simulink model "ChiefMaster_TTC580"  (R2022b)
settings: Solver=FixedStepAuto  StartTime=0.0  StopTime=10  FixedStep=0.01  RelTol=1e-3
values from neighbouring files (symbols this model uses):
  BattBox1_No = single(1)    [Parameters.m]
  BattBox2_No = single(2)    [Parameters.m]
  BattBox3_No = single(3)    [Parameters.m]
  CurrentLB = single(-3)    [Parameters.m]
  CurrentReductionConstant_Lvl0 = single(0.03)    [Parameters.m]
  CurrentReductionConstant_Lvl1 = single(0.05)    [Parameters.m]
  CurrentReductionConstant_Lvl2 = single(0.07)    [Parameters.m]
  CurrentReductionConstant_Lvl3 = single(0.1)    [Parameters.m]
  CurrentUB = single(3)    [Parameters.m]
  DCHV_Minus_In_Delay_ms = single(500)    [Parameters.m]
  FL_sHVC_CellBalanceVoltage_mV = single(3500)    [Parameters.m]
  FL_sInrushCurrent_dividebyzero = single(0.00001)    [Parameters.m]
  FL_u8HMI_BuzzerTimer = uint8(3)    [Parameters.m]
  IP_boActValue = true    [Parameters.m]
  IP_boDeactValue = false    [Parameters.m]
  IP_boInitValue = false    [Parameters.m]
  IP_s_LB = 18000    [Parameters.m]
  IP_s_UB = 22000    [Parameters.m]
  IP_sBatt1_ChargeCurrentMax_Factor = single(0.1)    [Parameters.m]
  IP_sBatt1_ChargeCurrentMax_LB = single(0)    [Parameters.m]
  IP_sBatt1_ChargeCurrentMax_Offset = single(0)    [Parameters.m]
  IP_sBatt1_ChargeCurrentMax_UB = single(6553.5)    [Parameters.m]
  IP_sBatt1_Current_Factor = single(0.1)    [Parameters.m]
  IP_sBatt1_Current_LB = single(-3276.8)    [Parameters.m]
  IP_sBatt1_Current_Offset = single(0)    [Parameters.m]
  IP_sBatt1_Current_UB = single(3276.8)    [Parameters.m]
  IP_sBatt1_DisChargeCurrentMax_Factor = single(0.1)    [Parameters.m]
  IP_sBatt1_DisChargeCurrentMax_LB = single(0)    [Parameters.m]
  IP_sBatt1_DisChargeCurrentMax_Offset = single(0)    [Parameters.m]
  IP_sBatt1_DisChargeCurrentMax_UB = single(6553.5)    [Parameters.m]
  IP_sBatt1_InsulationResistance_Factor = single(5)    [Parameters.m]
  IP_sBatt1_InsulationResistance_LB = single(0)    [Parameters.m]
  IP_sBatt1_InsulationResistance_Offset = single(0)    [Parameters.m]
  IP_sBatt1_InsulationResistance_UB = single(0)    [Parameters.m]
  IP_sBatt1_LiBa_IntResist_mOhm = single(25)    [Parameters.m]
  IP_sBatt1_SOC_Factor = single(1)    [Parameters.m]
  IP_sBatt1_SOC_LB = single(0)    [Parameters.m]
  IP_sBatt1_SOC_Offset = single(0)    [Parameters.m]
  IP_sBatt1_SOC_UB = single(100)    [Parameters.m]
  IP_sBatt1_SOH_Factor = single(1)    [Parameters.m]
  IP_sBatt1_SOH_LB = single(0)    [Parameters.m]
  IP_sBatt1_SOH_Offset = single(0)    [Parameters.m]
  IP_sBatt1_SOH_UB = single(100)    [Parameters.m]
  IP_sBatt1_Ubatt_Factor = single(0.1)    [Parameters.m]
  IP_sBatt1_Ubatt_LB = single(0)    [Parameters.m]
  IP_sBatt1_Ubatt_Offset = single(0)    [Parameters.m]
  IP_sBatt1_Ubatt_UB = single(6553.5)    [Parameters.m]
  IP_sBatt1_UserRi_Factor = single(1)    [Parameters.m]
  IP_sBatt1_UserRi_LB = single(0)    [Parameters.m]
  IP_sBatt1_UserRi_Offset = single(0)    [Parameters.m]
  IP_sBatt1_UserRi_UB = single(255)    [Parameters.m]
  IP_sBatt1_VoltageAtSensor_Factor = single(0.02)    [Parameters.m]
  IP_sBatt1_VoltageAtSensor_LB = single(0)    [Parameters.m]
  IP_sBatt1_VoltageAtSensor_Offset = single(0)    [Parameters.m]
  IP_sBatt1_VoltageAtSensor_UB = single(1310.7)    [Parameters.m]
  IP_sBatt2_LiBa_IntResist_mOhm = single(25)    [Parameters.m]
  IP_sBatt3_LiBa_IntResist_mOhm = single(25)    [Parameters.m]
  IP_sEM_LB = 2000    [Parameters.m]
  IP_sEM_UB = 8000    [Parameters.m]
  IP_sFB_LB = 5000    [Parameters.m]
  IP_sFB_UB = 10000    [Parameters.m]
  IP_sHVIL_LB = 12000    [Parameters.m]
  IP_sHVIL_UB = 15000    [Parameters.m]
  IP_sLoad_Voltage_Factor = single(1)    [Parameters.m]
  IP_sLoad_Voltage_LB = single(0)    [Parameters.m]
  IP_sLoad_Voltage_Offset = single(0)    [Parameters.m]
  IP_sLoad_Voltage_UB = single(65535)    [Parameters.m]
  IP_u8HVIL_Delay_ms = uint8(100)    [Parameters.m]
  IP_u8HW_IN_delay_ms = uint8(100)    [Parameters.m]
  IT_sInsulationSafeValue_kOhm = single(650)    [Parameters.m]
  IT_u8IMD_DelayTime_s = uint8(20)    [Parameters.m]
  MainHV_Minus_In_Delay = single(5)    [Parameters.m]
  MainHV_StatusDelay = single(5)    [Parameters.m]
  NotAvailable_uint16 = single(65535)    [Parameters.m]
  NotAvailable_uint8 = uint8(255)    [Parameters.m]
  OP_boHVIL_Supply = boolean(1)    [Parameters.m]
  SafeCurrentToCloseHV_A = single(5)    [Parameters.m]
  SafeVoltageToCloseHV_V = single(0.5)    [Parameters.m]
  UnexpectedBattChargingFcn_Available = boolean(1)    [Parameters.m]
  Voltage_NA_UB = uint16(65535)    [Parameters.m]
  VoltageSensorAvailableBB1 = boolean(0)    [Parameters.m]
  VoltageSensorAvailableBB2 = boolean(0)    [Parameters.m]
  VoltageSensorAvailableBB3 = boolean(0)    [Parameters.m]
libraries: simulink x184, Library_DataProcessing_v1_1 x167, Library_DataProcessing_v1 x142, libCM x28
(part 16 of 19)

== system ChiefMaster_TTC580/ChiefMaster/Input Processing/LiBa/LiBa_Box1/BMS_CellVoltageNumber/Subsystem2 ==
  byte2 : Inport
  C_LB_CellVoltage02_Timeout : Inport  Port=2
  Bus Creator : BusCreator  Inputs=3
  Constant : Constant  OutDataTypeStr=single
  Constant1 : Constant  Value=0  OutDataTypeStr=single
  Constant2 : Constant  Value=0  OutDataTypeStr=single
  Constant3 : Constant  Value=255  OutDataTypeStr=single
  Constant4 : Constant  Value=0  OutDataTypeStr=single
  Lib_InputProcessing+SafeValueSelector_Data : Library_DataProcessing_v1_1/Lib_InputProcessing+SafeValueSelector_Data  SystemSampleTime=-1  VariantActivationTime=update diagram  Latency=0  AutoFrameSizeCalculation=off
  IP_LB_BMS_ACT_Cel_V_Max_Cel_DataBus : Outport
  wires:
  C_LB_CellVoltage02_Timeout/1 -> Lib_InputProcessing+SafeValueSelector_Data/2
  Bus Creator/1 -> IP_LB_BMS_ACT_Cel_V_Max_Cel_DataBus/1  "IP_LB_BMS_ACT_Cel_V_Max_Cel_DataBus"
  Lib_InputProcessing+SafeValueSelector_Data/1 -> Bus Creator/1
  Constant/1 -> Lib_InputProcessing+SafeValueSelector_Data/3
  Constant4/1 -> Lib_InputProcessing+SafeValueSelector_Data/7, Lib_InputProcessing+SafeValueSelector_Data/8
  Lib_InputProcessing+SafeValueSelector_Data/2 -> Bus Creator/2
  Constant1/1 -> Lib_InputProcessing+SafeValueSelector_Data/4
  byte2/1 -> Lib_InputProcessing+SafeValueSelector_Data/1
  Lib_InputProcessing+SafeValueSelector_Data/3 -> Bus Creator/3
  Constant3/1 -> Lib_InputProcessing+SafeValueSelector_Data/6
  Constant2/1 -> Lib_InputProcessing+SafeValueSelector_Data/5

== system ChiefMaster_TTC580/ChiefMaster/Input Processing/LiBa/LiBa_Box1/BMS_CellVoltageNumber/Subsystem3 ==
  byte3 : Inport
  C_LB_CellVoltage02_Timeout : Inport  Port=2
  Bus Creator : BusCreator  Inputs=3
  Constant : Constant  OutDataTypeStr=single
  Constant1 : Constant  Value=0  OutDataTypeStr=single
  Constant2 : Constant  Value=0  OutDataTypeStr=single
  Constant3 : Constant  Value=255  OutDataTypeStr=single
  Constant4 : Constant  Value=0  OutDataTypeStr=single
  Lib_InputProcessing+SafeValueSelector_Data : Library_DataProcessing_v1_1/Lib_InputProcessing+SafeValueSelector_Data  SystemSampleTime=-1  VariantActivationTime=update diagram  Latency=0  AutoFrameSizeCalculation=off
  IP_LB_BMS_ACT_Cel_V_Max_CMU_DataBus : Outport
  wires:
  Constant2/1 -> Lib_InputProcessing+SafeValueSelector_Data/5
  Constant3/1 -> Lib_InputProcessing+SafeValueSelector_Data/6
  Lib_InputProcessing+SafeValueSelector_Data/3 -> Bus Creator/3
  byte3/1 -> Lib_InputProcessing+SafeValueSelector_Data/1
  Constant1/1 -> Lib_InputProcessing+SafeValueSelector_Data/4
  Lib_InputProcessing+SafeValueSelector_Data/2 -> Bus Creator/2
  Constant4/1 -> Lib_InputProcessing+SafeValueSelector_Data/8, Lib_InputProcessing+SafeValueSelector_Data/7
  Constant/1 -> Lib_InputProcessing+SafeValueSelector_Data/3
  Lib_InputProcessing+SafeValueSelector_Data/1 -> Bus Creator/1
  Bus Creator/1 -> IP_LB_BMS_ACT_Cel_V_Max_CMU_DataBus/1  "IP_LB_BMS_ACT_Cel_V_Max_CMU_DataBus"
  C_LB_CellVoltage02_Timeout/1 -> Lib_InputProcessing+SafeValueSelector_Data/2

== system ChiefMaster_TTC580/ChiefMaster/Input Processing/LiBa/LiBa_Box1/BMS_InsulationMonitor/Subsystem ==
  byte0 : Inport
  byte1 : Inport  Port=2
  C_LB_BMS_InsulationMonitor_Timeout : Inport  Port=3
  Bus Creator : BusCreator  Inputs=3
  Constant : Constant  OutDataTypeStr=single
  Constant1 : Constant  Value=0  OutDataTypeStr=single
  Constant2 : Constant  Value=0  OutDataTypeStr=single
  Constant3 : Constant  Value=65535  OutDataTypeStr=single
  Constant4 : Constant  Value=0  OutDataTypeStr=single
  Lib_2byte_ArthConcat : Library_DataProcessing_v1_1/Lib_2byte_ArthConcat  SystemSampleTime=-1  VariantActivationTime=update diagram  Latency=0  AutoFrameSizeCalculation=off
  Lib_InputProcessing+SafeValueSelector_Data : Library_DataProcessing_v1_1/Lib_InputProcessing+SafeValueSelector_Data  SystemSampleTime=-1  VariantActivationTime=update diagram  Latency=0  AutoFrameSizeCalculation=off
  IP_LB_BMS_Pack_Leak_Pos_Raw_mV_DataBus : Outport
  wires:
  Constant4/1 -> Lib_InputProcessing+SafeValueSelector_Data/7, Lib_InputProcessing+SafeValueSelector_Data/8
  Constant3/1 -> Lib_InputProcessing+SafeValueSelector_Data/6
  Constant2/1 -> Lib_InputProcessing+SafeValueSelector_Data/5
  Constant1/1 -> Lib_InputProcessing+SafeValueSelector_Data/4
  Constant/1 -> Lib_InputProcessing+SafeValueSelector_Data/3
  Bus Creator/1 -> IP_LB_BMS_Pack_Leak_Pos_Raw_mV_DataBus/1  "IP_LB_BMS_Pack_Leak_Pos_Raw_mV_DataBus"
  Lib_InputProcessing+SafeValueSelector_Data/3 -> Bus Creator/3
  Lib_InputProcessing+SafeValueSelector_Data/2 -> Bus Creator/2
  Lib_InputProcessing+SafeValueSelector_Data/1 -> Bus Creator/1
  C_LB_BMS_InsulationMonitor_Timeout/1 -> Lib_InputProcessing+SafeValueSelector_Data/2
  Lib_2byte_ArthConcat/1 -> Lib_InputProcessing+SafeValueSelector_Data/1
  byte1/1 -> Lib_2byte_ArthConcat/2
  byte0/1 -> Lib_2byte_ArthConcat/1

== system ChiefMaster_TTC580/ChiefMaster/Input Processing/LiBa/LiBa_Box1/BMS_InsulationMonitor/Subsystem1 ==
  byte2 : Inport
  byte3 : Inport  Port=2
  C_LB_BMS_InsulationMonitor_Timeout : Inport  Port=3
  Bus Creator : BusCreator  Inputs=3
  Constant : Constant  OutDataTypeStr=single
  Constant1 : Constant  Value=0  OutDataTypeStr=single
  Constant2 : Constant  Value=0  OutDataTypeStr=single
  Constant3 : Constant  Value=65535  OutDataTypeStr=single
  Constant4 : Constant  Value=0  OutDataTypeStr=single
  Lib_2byte_ArthConcat : Library_DataProcessing_v1_1/Lib_2byte_ArthConcat  SystemSampleTime=-1  VariantActivationTime=update diagram  Latency=0  AutoFrameSizeCalculation=off
  Lib_InputProcessing+SafeValueSelector_Data : Library_DataProcessing_v1_1/Lib_InputProcessing+SafeValueSelector_Data  SystemSampleTime=-1  VariantActivationTime=update diagram  Latency=0  AutoFrameSizeCalculation=off
  IP_LB_BMS_Pack_Leak_Neg_Raw_mV_DataBus : Outport
  wires:
  Bus Creator/1 -> IP_LB_BMS_Pack_Leak_Neg_Raw_mV_DataBus/1  "IP_LB_BMS_Pack_Leak_Neg_Raw_mV_DataBus"
  C_LB_BMS_InsulationMonitor_Timeout/1 -> Lib_InputProcessing+SafeValueSelector_Data/2
  byte3/1 -> Lib_2byte_ArthConcat/2
  byte2/1 -> Lib_2byte_ArthConcat/1
  Constant3/1 -> Lib_InputProcessing+SafeValueSelector_Data/6
  Constant2/1 -> Lib_InputProcessing+SafeValueSelector_Data/5
  Lib_InputProcessing+SafeValueSelector_Data/3 -> Bus Creator/3
  Lib_InputProcessing+SafeValueSelector_Data/2 -> Bus Creator/2
  Constant/1 -> Lib_InputProcessing+SafeValueSelector_Data/3
  Lib_InputProcessing+SafeValueSelector_Data/1 -> Bus Creator/1
  Constant1/1 -> Lib_InputProcessing+SafeValueSelector_Data/4
  Lib_2byte_ArthConcat/1 -> Lib_InputProcessing+SafeValueSelector_Data/1
  Constant4/1 -> Lib_InputProcessing+SafeValueSelector_Data/7, Lib_InputProcessing+SafeValueSelector_Data/8

== system ChiefMaster_TTC580/ChiefMaster/Input Processing/LiBa/LiBa_Box1/BMS_InsulationMonitor/Subsystem2 ==
  byte4 : Inport
  byte5 : Inport  Port=2
  C_LB_BMS_InsulationMonitor_Timeout : Inport  Port=3
  Bus Creator : BusCreator  Inputs=3
  Constant : Constant  OutDataTypeStr=single
  Constant1 : Constant  Value=0  OutDataTypeStr=single
  Constant2 : Constant  Value=0  OutDataTypeStr=single
  Constant3 : Constant  Value=65535  OutDataTypeStr=single
  Constant4 : Constant  Value=0  OutDataTypeStr=single
  Lib_2byte_ArthConcat : Library_DataProcessing_v1_1/Lib_2byte_ArthConcat  SystemSampleTime=-1  VariantActivationTime=update diagram  Latency=0  AutoFrameSizeCalculation=off
  Lib_InputProcessing+SafeValueSelector_Data : Library_DataProcessing_v1_1/Lib_InputProcessing+SafeValueSelector_Data  SystemSampleTime=-1  VariantActivationTime=update diagram  Latency=0  AutoFrameSizeCalculation=off
  IP_LB_BMS_Pack_Leak_Mid_Raw_mV_DataBus : Outport
  wires:
  byte5/1 -> Lib_2byte_ArthConcat/2
  byte4/1 -> Lib_2byte_ArthConcat/1
  C_LB_BMS_InsulationMonitor_Timeout/1 -> Lib_InputProcessing+SafeValueSelector_Data/2
  Bus Creator/1 -> IP_LB_BMS_Pack_Leak_Mid_Raw_mV_DataBus/1  "IP_LB_BMS_Pack_Leak_Mid_Raw_mV_DataBus"
  Lib_InputProcessing+SafeValueSelector_Data/1 -> Bus Creator/1
  Constant/1 -> Lib_InputProcessing+SafeValueSelector_Data/3
  Constant4/1 -> Lib_InputProcessing+SafeValueSelector_Data/7, Lib_InputProcessing+SafeValueSelector_Data/8
  Lib_InputProcessing+SafeValueSelector_Data/2 -> Bus Creator/2
  Constant1/1 -> Lib_InputProcessing+SafeValueSelector_Data/4
  Lib_2byte_ArthConcat/1 -> Lib_InputProcessing+SafeValueSelector_Data/1
  Lib_InputProcessing+SafeValueSelector_Data/3 -> Bus Creator/3
  Constant3/1 -> Lib_InputProcessing+SafeValueSelector_Data/6
  Constant2/1 -> Lib_InputProcessing+SafeValueSelector_Data/5

== system ChiefMaster_TTC580/ChiefMaster/Input Processing/LiBa/LiBa_Box1/BMS_Status01/Subsystem1 ==
  byte1 : Inport
  C_LB_BMS_Status01_Timeout : Inport  Port=2
  Bus Creator : BusCreator  Inputs=3
  Constant : Constant  OutDataTypeStr=single
  Constant1 : Constant  Value=0  OutDataTypeStr=single
  Constant2 : Constant  Value=0  OutDataTypeStr=single
  Constant3 : Constant  Value=255  OutDataTypeStr=single
  Constant4 : Constant  Value=0  OutDataTypeStr=single
  Lib_InputProcessing+SafeValueSelector_Data : Library_DataProcessing_v1_1/Lib_InputProcessing+SafeValueSelector_Data  SystemSampleTime=-1  VariantActivationTime=update diagram  Latency=0  AutoFrameSizeCalculation=off
  IP_LB_BMS_IO_state_Input_DataBus : Outport
  wires:
  byte1/1 -> Lib_InputProcessing+SafeValueSelector_Data/1
  Bus Creator/1 -> IP_LB_BMS_IO_state_Input_DataBus/1  "IP_LB_BMS_IO_state_Input_DataBus"
  C_LB_BMS_Status01_Timeout/1 -> Lib_InputProcessing+SafeValueSelector_Data/2
  Constant3/1 -> Lib_InputProcessing+SafeValueSelector_Data/6
  Constant2/1 -> Lib_InputProcessing+SafeValueSelector_Data/5
  Lib_InputProcessing+SafeValueSelector_Data/3 -> Bus Creator/3
  Lib_InputProcessing+SafeValueSelector_Data/2 -> Bus Creator/2
  Constant/1 -> Lib_InputProcessing+SafeValueSelector_Data/3
  Lib_InputProcessing+SafeValueSelector_Data/1 -> Bus Creator/1
  Constant1/1 -> Lib_InputProcessing+SafeValueSelector_Data/4
  Constant4/1 -> Lib_InputProcessing+SafeValueSelector_Data/7, Lib_InputProcessing+SafeValueSelector_Data/8

== system ChiefMaster_TTC580/ChiefMaster/Input Processing/LiBa/LiBa_Box1/BMS_Status01/Subsystem2 ==
  byte2 : Inport
  C_LB_BMS_Status01_Timeout : Inport  Port=2
  Bus Creator : BusCreator  Inputs=3
  Constant : Constant  OutDataTypeStr=single
  Constant1 : Constant  Value=0  OutDataTypeStr=single
  Constant2 : Constant  Value=0  OutDataTypeStr=single
  Constant3 : Constant  Value=255  OutDataTypeStr=single
  Constant4 : Constant  Value=0  OutDataTypeStr=single
  Lib_InputProcessing+SafeValueSelector_Data : Library_DataProcessing_v1_1/Lib_InputProcessing+SafeValueSelector_Data  SystemSampleTime=-1  VariantActivationTime=update diagram  Latency=0  AutoFrameSizeCalculation=off
  IP_LB_BMS_IO_State_Output_DataBus : Outport
  wires:
  byte2/1 -> Lib_InputProcessing+SafeValueSelector_Data/1
  C_LB_BMS_Status01_Timeout/1 -> Lib_InputProcessing+SafeValueSelector_Data/2
  Bus Creator/1 -> IP_LB_BMS_IO_State_Output_DataBus/1  "IP_LB_BMS_IO_State_Output_DataBus"
  Lib_InputProcessing+SafeValueSelector_Data/1 -> Bus Creator/1
  Constant/1 -> Lib_InputProcessing+SafeValueSelector_Data/3
  Constant4/1 -> Lib_InputProcessing+SafeValueSelector_Data/7, Lib_InputProcessing+SafeValueSelector_Data/8
  Lib_InputProcessing+SafeValueSelector_Data/2 -> Bus Creator/2
  Constant1/1 -> Lib_InputProcessing+SafeValueSelector_Data/4
  Lib_InputProcessing+SafeValueSelector_Data/3 -> Bus Creator/3
  Constant3/1 -> Lib_InputProcessing+SafeValueSelector_Data/6
  Constant2/1 -> Lib_InputProcessing+SafeValueSelector_Data/5

== system ChiefMaster_TTC580/ChiefMaster/Input Processing/LiBa/LiBa_Box1/BMS_Status01/Subsystem3 ==
  byte4 : Inport
  byte5 : Inport  Port=2
  C_LB_BMS_Status01_Timeout : Inport  Port=3
  Bus Creator : BusCreator  Inputs=3
  Constant : Constant  Value=0.1  OutDataTypeStr=single
  Constant1 : Constant  Value=0  OutDataTypeStr=single
  Constant2 : Constant  Value=0  OutDataTypeStr=single
  Constant3 : Constant  Value=6553.5  OutDataTypeStr=single
  Constant4 : Constant  Value=0  OutDataTypeStr=single
  Lib_2byte_ArthConcat : Library_DataProcessing_v1_1/Lib_2byte_ArthConcat  SystemSampleTime=-1  VariantActivationTime=update diagram  Latency=0  AutoFrameSizeCalculation=off
  Lib_InputProcessing+SafeValueSelector_Data : Library_DataProcessing_v1_1/Lib_InputProcessing+SafeValueSelector_Data  SystemSampleTime=-1  VariantActivationTime=update diagram  Latency=0  AutoFrameSizeCalculation=off
  IP_LB_BMS_DYN_Lim_Current_IN_A_DataBus : Outport
  wires:
  Bus Creator/1 -> IP_LB_BMS_DYN_Lim_Current_IN_A_DataBus/1  "IP_LB_BMS_DYN_Lim_Current_IN_A_DataBus"
  Constant3/1 -> Lib_InputProcessing+SafeValueSelector_Data/6
  Lib_2byte_ArthConcat/1 -> Lib_InputProcessing+SafeValueSelector_Data/1
  Constant1/1 -> Lib_InputProcessing+SafeValueSelector_Data/4
  Constant4/1 -> Lib_InputProcessing+SafeValueSelector_Data/8, Lib_InputProcessing+SafeValueSelector_Data/7
  Constant/1 -> Lib_InputProcessing+SafeValueSelector_Data/3
  Constant2/1 -> Lib_InputProcessing+SafeValueSelector_Data/5
  Lib_InputProcessing+SafeValueSelector_Data/1 -> Bus Creator/1
  Lib_InputProcessing+SafeValueSelector_Data/3 -> Bus Creator/3
  Lib_InputProcessing+SafeValueSelector_Data/2 -> Bus Creator/2
  byte4/1 -> Lib_2byte_ArthConcat/1
  byte5/1 -> Lib_2byte_ArthConcat/2
  C_LB_BMS_Status01_Timeout/1 -> Lib_InputProcessing+SafeValueSelector_Data/2

== system ChiefMaster_TTC580/ChiefMaster/Input Processing/LiBa/LiBa_Box1/BMS_Status01/Subsystem4 ==
  byte6 : Inport
  byte7 : Inport  Port=2
  C_LB_BMS_Status01_Timeout : Inport  Port=3
  Bus Creator : BusCreator  Inputs=3
  Constant : Constant  Value=0.1  OutDataTypeStr=single
  Constant1 : Constant  Value=0  OutDataTypeStr=single
  Constant2 : Constant  Value=0  OutDataTypeStr=single
  Constant3 : Constant  Value=6553.5  OutDataTypeStr=single
  Constant4 : Constant  Value=0  OutDataTypeStr=single
  Lib_2byte_ArthConcat : Library_DataProcessing_v1_1/Lib_2byte_ArthConcat  SystemSampleTime=-1  VariantActivationTime=update diagram  Latency=0  AutoFrameSizeCalculation=off
  Lib_InputProcessing+SafeValueSelector_Data : Library_DataProcessing_v1_1/Lib_InputProcessing+SafeValueSelector_Data  SystemSampleTime=-1  VariantActivationTime=update diagram  Latency=0  AutoFrameSizeCalculation=off
  IP_LB_BMS_DYN_Lim_Current_OUT_A_DataBus : Outport
  wires:
  C_LB_BMS_Status01_Timeout/1 -> Lib_InputProcessing+SafeValueSelector_Data/2
  byte7/1 -> Lib_2byte_ArthConcat/2
  byte6/1 -> Lib_2byte_ArthConcat/1
  Lib_InputProcessing+SafeValueSelector_Data/2 -> Bus Creator/2
  Lib_InputProcessing+SafeValueSelector_Data/3 -> Bus Creator/3
  Lib_InputProcessing+SafeValueSelector_Data/1 -> Bus Creator/1
  Constant2/1 -> Lib_InputProcessing+SafeValueSelector_Data/5
  Constant/1 -> Lib_InputProcessing+SafeValueSelector_Data/3
  Constant4/1 -> Lib_InputProcessing+SafeValueSelector_Data/7, Lib_InputProcessing+SafeValueSelector_Data/8
  Constant1/1 -> Lib_InputProcessing+SafeValueSelector_Data/4
  Lib_2byte_ArthConcat/1 -> Lib_InputProcessing+SafeValueSelector_Data/1
  Constant3/1 -> Lib_InputProcessing+SafeValueSelector_Data/6
  Bus Creator/1 -> IP_LB_BMS_DYN_Lim_Current_OUT_A_DataBus/1  "IP_LB_BMS_DYN_Lim_Current_OUT_A_DataBus"

== system ChiefMaster_TTC580/ChiefMaster/Input Processing/LiBa/LiBa_Box1/BMS_Status02/Subsystem1 ==
  byte2 : Inport
  byte3 : Inport  Port=2
  byte4 : Inport  Port=3
  byte5 : Inport  Port=4
  C_LB_BMS_Status02_Timeout : Inport  Port=5
  Bus Creator : BusCreator  Inputs=3
  Constant : Constant  Value=0.01  OutDataTypeStr=single
  Constant1 : Constant  Value=0  OutDataTypeStr=single
  Constant2 : Constant  Value=-21474836.48  OutDataTypeStr=single
  Constant3 : Constant  Value=21474836.47  OutDataTypeStr=single
  Constant4 : Constant  Value=0  OutDataTypeStr=single
  Data Type Conversion : DataTypeConversion  OutDataTypeStr=int32  SaturateOnIntegerOverflow=off  RndMeth=Floor
  Lib_4byte_ArthConcat : Library_DataProcessing_v1_1/Lib_4byte_ArthConcat  SystemSampleTime=-1  VariantActivationTime=update diagram  Latency=0  AutoFrameSizeCalculation=off
  Lib_InputProcessing+SafeValueSelector_Data : Library_DataProcessing_v1_1/Lib_InputProcessing+SafeValueSelector_Data  SystemSampleTime=-1  VariantActivationTime=update diagram  Latency=0  AutoFrameSizeCalculation=off
  IP_LB_BMS_Pack_Current_Master_mA_DataBus : Outport
  wires:
  Data Type Conversion/1 -> Lib_InputProcessing+SafeValueSelector_Data/1
  Bus Creator/1 -> IP_LB_BMS_Pack_Current_Master_mA_DataBus/1  "IP_LB_BMS_Pack_Current_Master_mA_DataBus"
  Constant3/1 -> Lib_InputProcessing+SafeValueSelector_Data/6
  Lib_4byte_ArthConcat/1 -> Data Type Conversion/1
  Constant1/1 -> Lib_InputProcessing+SafeValueSelector_Data/4
  Constant4/1 -> Lib_InputProcessing+SafeValueSelector_Data/8, Lib_InputProcessing+SafeValueSelector_Data/7
  Constant/1 -> Lib_InputProcessing+SafeValueSelector_Data/3
  Constant2/1 -> Lib_InputProcessing+SafeValueSelector_Data/5
  Lib_InputProcessing+SafeValueSelector_Data/1 -> Bus Creator/1
  Lib_InputProcessing+SafeValueSelector_Data/3 -> Bus Creator/3
  Lib_InputProcessing+SafeValueSelector_Data/2 -> Bus Creator/2
  byte2/1 -> Lib_4byte_ArthConcat/1
  byte3/1 -> Lib_4byte_ArthConcat/2
  C_LB_BMS_Status02_Timeout/1 -> Lib_InputProcessing+SafeValueSelector_Data/2
  byte4/1 -> Lib_4byte_ArthConcat/3
  byte5/1 -> Lib_4byte_ArthConcat/4

== system ChiefMaster_TTC580/ChiefMaster/Input Processing/LiBa/LiBa_Box1/BMS_Status02/Subsystem2 ==
  byte6 : Inport
  byte7 : Inport  Port=2
  C_LB_BMS_Status02_Timeout : Inport  Port=3
  Bus Creator : BusCreator  Inputs=3
  Constant : Constant  Value=0.1  OutDataTypeStr=single
  Constant1 : Constant  Value=0  OutDataTypeStr=single
  Constant2 : Constant  Value=0  OutDataTypeStr=single
  Constant3 : Constant  Value=6553.5  OutDataTypeStr=single
  Constant4 : Constant  Value=0  OutDataTypeStr=single
  Lib_2byte_ArthConcat : Library_DataProcessing_v1_1/Lib_2byte_ArthConcat  SystemSampleTime=-1  VariantActivationTime=update diagram  Latency=0  AutoFrameSizeCalculation=off
  Lib_InputProcessing+SafeValueSelector_Data : Library_DataProcessing_v1_1/Lib_InputProcessing+SafeValueSelector_Data  SystemSampleTime=-1  VariantActivationTime=update diagram  Latency=0  AutoFrameSizeCalculation=off
  IP_LB_BMS_Pack_V_Cells_DataBus : Outport
  wires:
  Lib_2byte_ArthConcat/1 -> Lib_InputProcessing+SafeValueSelector_Data/1
  Bus Creator/1 -> IP_LB_BMS_Pack_V_Cells_DataBus/1  "IP_LB_BMS_Pack_V_Cells_DataBus"
  Constant3/1 -> Lib_InputProcessing+SafeValueSelector_Data/6
  Constant1/1 -> Lib_InputProcessing+SafeValueSelector_Data/4
  Constant4/1 -> Lib_InputProcessing+SafeValueSelector_Data/8, Lib_InputProcessing+SafeValueSelector_Data/7
  Constant/1 -> Lib_InputProcessing+SafeValueSelector_Data/3
  Constant2/1 -> Lib_InputProcessing+SafeValueSelector_Data/5
  Lib_InputProcessing+SafeValueSelector_Data/1 -> Bus Creator/1
  Lib_InputProcessing+SafeValueSelector_Data/3 -> Bus Creator/3
  Lib_InputProcessing+SafeValueSelector_Data/2 -> Bus Creator/2
  byte6/1 -> Lib_2byte_ArthConcat/1
  byte7/1 -> Lib_2byte_ArthConcat/2
  C_LB_BMS_Status02_Timeout/1 -> Lib_InputProcessing+SafeValueSelector_Data/2

== system ChiefMaster_TTC580/ChiefMaster/Input Processing/LiBa/LiBa_Box1/BMS_Status02/Subsystem3 ==
  byte0 : Inport
  byte1 : Inport  Port=2
  C_LB_BMS_Status02_Timeout : Inport  Port=3
  Bus Creator : BusCreator  Inputs=3
  Constant : Constant  Value=0.01  OutDataTypeStr=single
  Constant1 : Constant  Value=0  OutDataTypeStr=single
  Constant2 : Constant  Value=-327.68  OutDataTypeStr=single
  Constant3 : Constant  Value=327.67  OutDataTypeStr=single
  Constant4 : Constant  Value=0  OutDataTypeStr=single
  Data Type Conversion : DataTypeConversion  OutDataTypeStr=int16  SaturateOnIntegerOverflow=off  RndMeth=Floor
  Lib_2byte_ArthConcat : Library_DataProcessing_v1_1/Lib_2byte_ArthConcat  SystemSampleTime=-1  VariantActivationTime=update diagram  Latency=0  AutoFrameSizeCalculation=off
  Lib_InputProcessing+SafeValueSelector_Data : Library_DataProcessing_v1_1/Lib_InputProcessing+SafeValueSelector_Data  SystemSampleTime=-1  VariantActivationTime=update diagram  Latency=0  AutoFrameSizeCalculation=off
  IP_LB_BMS_Pack_Q_SOC_Internal_DataBus : Outport
  wires:
  C_LB_BMS_Status02_Timeout/1 -> Lib_InputProcessing+SafeValueSelector_Data/2
  byte1/1 -> Lib_2byte_ArthConcat/2
  byte0/1 -> Lib_2byte_ArthConcat/1
  Lib_InputProcessing+SafeValueSelector_Data/2 -> Bus Creator/2
  Lib_InputProcessing+SafeValueSelector_Data/3 -> Bus Creator/3
  Lib_InputProcessing+SafeValueSelector_Data/1 -> Bus Creator/1
  Constant2/1 -> Lib_InputProcessing+SafeValueSelector_Data/5
  Constant/1 -> Lib_InputProcessing+SafeValueSelector_Data/3
  Constant4/1 -> Lib_InputProcessing+SafeValueSelector_Data/7, Lib_InputProcessing+SafeValueSelector_Data/8
  Constant1/1 -> Lib_InputProcessing+SafeValueSelector_Data/4
  Lib_2byte_ArthConcat/1 -> Data Type Conversion/1
  Constant3/1 -> Lib_InputProcessing+SafeValueSelector_Data/6
  Bus Creator/1 -> IP_LB_BMS_Pack_Q_SOC_Internal_DataBus/1  "IP_LB_BMS_Pack_Q_SOC_Internal_DataBus"
  Data Type Conversion/1 -> Lib_InputProcessing+SafeValueSelector_Data/1

== system ChiefMaster_TTC580/ChiefMaster/Input Processing/LiBa/LiBa_Box1/BMS_Status03/Subsystem3 ==
  byte0 : Inport
  byte1 : Inport  Port=2
  C_LB_BMS_Status03_Timeout : Inport  Port=3
  Bus Creator : BusCreator  Inputs=3
  Constant : Constant  Value=0.1  OutDataTypeStr=single
  Constant1 : Constant  Value=0  OutDataTypeStr=single
  Constant2 : Constant  Value=0  OutDataTypeStr=single
  Constant3 : Constant  Value=6553.5  OutDataTypeStr=single
  Constant4 : Constant  Value=0  OutDataTypeStr=single
  Lib_2byte_ArthConcat : Library_DataProcessing_v1_1/Lib_2byte_ArthConcat  SystemSampleTime=-1  VariantActivationTime=update diagram  Latency=0  AutoFrameSizeCalculation=off
  Lib_InputProcessing+SafeValueSelector_Data : Library_DataProcessing_v1_1/Lib_InputProcessing+SafeValueSelector_Data  SystemSampleTime=-1  VariantActivationTime=update diagram  Latency=0  AutoFrameSizeCalculation=off
  IP_LB_BMS_REQ_Charger_Current_A_DataBus : Outport
  wires:
  Lib_2byte_ArthConcat/1 -> Lib_InputProcessing+SafeValueSelector_Data/1
  Bus Creator/1 -> IP_LB_BMS_REQ_Charger_Current_A_DataBus/1  "IP_LB_BMS_REQ_Charger_Current_A_DataBus"
  Constant3/1 -> Lib_InputProcessing+SafeValueSelector_Data/6
  Constant1/1 -> Lib_InputProcessing+SafeValueSelector_Data/4
  Constant4/1 -> Lib_InputProcessing+SafeValueSelector_Data/8, Lib_InputProcessing+SafeValueSelector_Data/7
  Constant/1 -> Lib_InputProcessing+SafeValueSelector_Data/3
  Constant2/1 -> Lib_InputProcessing+SafeValueSelector_Data/5
  Lib_InputProcessing+SafeValueSelector_Data/1 -> Bus Creator/1
  Lib_InputProcessing+SafeValueSelector_Data/3 -> Bus Creator/3
  Lib_InputProcessing+SafeValueSelector_Data/2 -> Bus Creator/2
  byte0/1 -> Lib_2byte_ArthConcat/1
  byte1/1 -> Lib_2byte_ArthConcat/2
  C_LB_BMS_Status03_Timeout/1 -> Lib_InputProcessing+SafeValueSelector_Data/2

== system ChiefMaster_TTC580/ChiefMaster/Input Processing/LiBa/LiBa_Box2/BMS_CellTemperature/Subsystem ==
  byte0 : Inport
  C_LB_BMS_CellTemperature_Timeout : Inport  Port=2
  Bus Creator : BusCreator  Inputs=3
  Constant : Constant  OutDataTypeStr=single
  Constant1 : Constant  Value=0  OutDataTypeStr=single
  Constant2 : Constant  Value=-128  OutDataTypeStr=single
  Constant3 : Constant  Value=127  OutDataTypeStr=single
  Constant4 : Constant  Value=0  OutDataTypeStr=single
  Data Type Conversion : DataTypeConversion  OutDataTypeStr=int8  SaturateOnIntegerOverflow=off  RndMeth=Floor
  Lib_InputProcessing+SafeValueSelector_Data : Library_DataProcessing_v1_1/Lib_InputProcessing+SafeValueSelector_Data  SystemSampleTime=-1  VariantActivationTime=update diagram  Latency=0  AutoFrameSizeCalculation=off
  IP_LB_BMS_ACT_Cel_T_Avg_DataBus : Outport
  wires:
  byte0/1 -> Data Type Conversion/1
  C_LB_BMS_CellTemperature_Timeout/1 -> Lib_InputProcessing+SafeValueSelector_Data/2
  Lib_InputProcessing+SafeValueSelector_Data/1 -> Bus Creator/1
  Lib_InputProcessing+SafeValueSelector_Data/2 -> Bus Creator/2
  Lib_InputProcessing+SafeValueSelector_Data/3 -> Bus Creator/3
  Bus Creator/1 -> IP_LB_BMS_ACT_Cel_T_Avg_DataBus/1  "IP_LB_BMS_ACT_Cel_T_Avg_DataBus"
  Constant/1 -> Lib_InputProcessing+SafeValueSelector_Data/3
  Constant1/1 -> Lib_InputProcessing+SafeValueSelector_Data/4
  Constant2/1 -> Lib_InputProcessing+SafeValueSelector_Data/5
  Constant3/1 -> Lib_InputProcessing+SafeValueSelector_Data/6
  Constant4/1 -> Lib_InputProcessing+SafeValueSelector_Data/8, Lib_InputProcessing+SafeValueSelector_Data/7
  Data Type Conversion/1 -> Lib_InputProcessing+SafeValueSelector_Data/1

== system ChiefMaster_TTC580/ChiefMaster/Input Processing/LiBa/LiBa_Box2/BMS_CellTemperature/Subsystem1 ==
  byte1 : Inport
  C_LB_BMS_CellTemperature_Timeout : Inport  Port=2
  Bus Creator : BusCreator  Inputs=3
  Constant : Constant  OutDataTypeStr=single
  Constant1 : Constant  Value=0  OutDataTypeStr=single
  Constant2 : Constant  Value=-128  OutDataTypeStr=single
  Constant3 : Constant  Value=127  OutDataTypeStr=single
  Constant4 : Constant  Value=0  OutDataTypeStr=single
  Data Type Conversion : DataTypeConversion  OutDataTypeStr=int8  SaturateOnIntegerOverflow=off  RndMeth=Floor
  Lib_InputProcessing+SafeValueSelector_Data : Library_DataProcessing_v1_1/Lib_InputProcessing+SafeValueSelector_Data  SystemSampleTime=-1  VariantActivationTime=update diagram  Latency=0  AutoFrameSizeCalculation=off
  IP_LB_BMS_ACT_Cel_T_Min_Value_DataBus : Outport
  wires:
  Constant4/1 -> Lib_InputProcessing+SafeValueSelector_Data/8, Lib_InputProcessing+SafeValueSelector_Data/7
  byte1/1 -> Data Type Conversion/1
  Constant1/1 -> Lib_InputProcessing+SafeValueSelector_Data/4
  Lib_InputProcessing+SafeValueSelector_Data/1 -> Bus Creator/1
  Constant/1 -> Lib_InputProcessing+SafeValueSelector_Data/3
  Lib_InputProcessing+SafeValueSelector_Data/2 -> Bus Creator/2
  Lib_InputProcessing+SafeValueSelector_Data/3 -> Bus Creator/3
  Constant2/1 -> Lib_InputProcessing+SafeValueSelector_Data/5
  Constant3/1 -> Lib_InputProcessing+SafeValueSelector_Data/6
  C_LB_BMS_CellTemperature_Timeout/1 -> Lib_InputProcessing+SafeValueSelector_Data/2
  Bus Creator/1 -> IP_LB_BMS_ACT_Cel_T_Min_Value_DataBus/1  "IP_LB_BMS_ACT_Cel_T_Min_Value_DataBus"
  Data Type Conversion/1 -> Lib_InputProcessing+SafeValueSelector_Data/1

== system ChiefMaster_TTC580/ChiefMaster/Input Processing/LiBa/LiBa_Box2/BMS_CellTemperature/Subsystem2 ==
  byte2 : Inport
  C_LB_BMS_CellTemperature_Timeout : Inport  Port=2
  Bus Creator : BusCreator  Inputs=3
  Constant : Constant  OutDataTypeStr=single
  Constant1 : Constant  Value=0  OutDataTypeStr=single
  Constant2 : Constant  Value=-128  OutDataTypeStr=single
  Constant3 : Constant  Value=127  OutDataTypeStr=single
  Constant4 : Constant  Value=0  OutDataTypeStr=single
  Data Type Conversion : DataTypeConversion  OutDataTypeStr=int8  SaturateOnIntegerOverflow=off  RndMeth=Floor
  Lib_InputProcessing+SafeValueSelector_Data : Library_DataProcessing_v1_1/Lib_InputProcessing+SafeValueSelector_Data  SystemSampleTime=-1  VariantActivationTime=update diagram  Latency=0  AutoFrameSizeCalculation=off
  IP_LB_BMS_ACT_Cel_T_Max_Value_DataBus : Outport
  wires:
  Constant2/1 -> Lib_InputProcessing+SafeValueSelector_Data/5
  Constant3/1 -> Lib_InputProcessing+SafeValueSelector_Data/6
  Lib_InputProcessing+SafeValueSelector_Data/3 -> Bus Creator/3
  byte2/1 -> Data Type Conversion/1
  Constant1/1 -> Lib_InputProcessing+SafeValueSelector_Data/4
  Lib_InputProcessing+SafeValueSelector_Data/2 -> Bus Creator/2
  Constant4/1 -> Lib_InputProcessing+SafeValueSelector_Data/8, Lib_InputProcessing+SafeValueSelector_Data/7
  Constant/1 -> Lib_InputProcessing+SafeValueSelector_Data/3
  Lib_InputProcessing+SafeValueSelector_Data/1 -> Bus Creator/1
  Bus Creator/1 -> IP_LB_BMS_ACT_Cel_T_Max_Value_DataBus/1  "IP_LB_BMS_ACT_Cel_T_Max_Value_DataBus"
  C_LB_BMS_CellTemperature_Timeout/1 -> Lib_InputProcessing+SafeValueSelector_Data/2
  Data Type Conversion/1 -> Lib_InputProcessing+SafeValueSelector_Data/1

== system ChiefMaster_TTC580/ChiefMaster/Input Processing/LiBa/LiBa_Box2/BMS_CellTemperature/Subsystem3 ==
  byte3 : Inport
  C_LB_BMS_CellTemperature_Timeout : Inport  Port=2
  Bus Creator : BusCreator  Inputs=3
  Constant : Constant  OutDataTypeStr=single
  Constant1 : Constant  Value=0  OutDataTypeStr=single
  Constant2 : Constant  Value=0  OutDataTypeStr=single
  Constant3 : Constant  Value=255  OutDataTypeStr=single
  Constant4 : Constant  Value=0  OutDataTypeStr=single
  Lib_InputProcessing+SafeValueSelector_Data : Library_DataProcessing_v1_1/Lib_InputProcessing+SafeValueSelector_Data  SystemSampleTime=-1  VariantActivationTime=update diagram  Latency=0  AutoFrameSizeCalculation=off
  IP_LB_BMS_ACT_Cel_T_Min_Cel_DataBus : Outport
  wires:
  C_LB_BMS_CellTemperature_Timeout/1 -> Lib_InputProcessing+SafeValueSelector_Data/2
  Bus Creator/1 -> IP_LB_BMS_ACT_Cel_T_Min_Cel_DataBus/1  "IP_LB_BMS_ACT_Cel_T_Min_Cel_DataBus"
  Lib_InputProcessing+SafeValueSelector_Data/1 -> Bus Creator/1
  Constant/1 -> Lib_InputProcessing+SafeValueSelector_Data/3
  Constant4/1 -> Lib_InputProcessing+SafeValueSelector_Data/7, Lib_InputProcessing+SafeValueSelector_Data/8
  Lib_InputProcessing+SafeValueSelector_Data/2 -> Bus Creator/2
  Constant1/1 -> Lib_InputProcessing+SafeValueSelector_Data/4
  byte3/1 -> Lib_InputProcessing+SafeValueSelector_Data/1
  Lib_InputProcessing+SafeValueSelector_Data/3 -> Bus Creator/3
  Constant3/1 -> Lib_InputProcessing+SafeValueSelector_Data/6
  Constant2/1 -> Lib_InputProcessing+SafeValueSelector_Data/5

== system ChiefMaster_TTC580/ChiefMaster/Input Processing/LiBa/LiBa_Box2/BMS_CellTemperature/Subsystem4 ==
  byte1 : Inport
  C_LB_BMS_CellTemperature_Timeout : Inport  Port=2
  Bus Creator : BusCreator  Inputs=3
  Constant : Constant  OutDataTypeStr=single
  Constant1 : Constant  Value=0  OutDataTypeStr=single
  Constant2 : Constant  Value=0  OutDataTypeStr=single
  Constant3 : Constant  Value=255  OutDataTypeStr=single
  Constant4 : Constant  Value=0  OutDataTypeStr=single
  Lib_InputProcessing+SafeValueSelector_Data : Library_DataProcessing_v1_1/Lib_InputProcessing+SafeValueSelector_Data  SystemSampleTime=-1  VariantActivationTime=update diagram  Latency=0  AutoFrameSizeCalculation=off
  IP_LB_BMS_ACT_Cel_T_Min_CMU_DataBus : Outport
  wires:
  Bus Creator/1 -> IP_LB_BMS_ACT_Cel_T_Min_CMU_DataBus/1  "IP_LB_BMS_ACT_Cel_T_Min_CMU_DataBus"
  C_LB_BMS_CellTemperature_Timeout/1 -> Lib_InputProcessing+SafeValueSelector_Data/2
  Constant3/1 -> Lib_InputProcessing+SafeValueSelector_Data/6
  Constant2/1 -> Lib_InputProcessing+SafeValueSelector_Data/5
  Lib_InputProcessing+SafeValueSelector_Data/3 -> Bus Creator/3
  Lib_InputProcessing+SafeValueSelector_Data/2 -> Bus Creator/2
  Constant/1 -> Lib_InputProcessing+SafeValueSelector_Data/3
  Lib_InputProcessing+SafeValueSelector_Data/1 -> Bus Creator/1
  Constant1/1 -> Lib_InputProcessing+SafeValueSelector_Data/4
  byte1/1 -> Lib_InputProcessing+SafeValueSelector_Data/1
  Constant4/1 -> Lib_InputProcessing+SafeValueSelector_Data/7, Lib_InputProcessing+SafeValueSelector_Data/8

== system ChiefMaster_TTC580/ChiefMaster/Input Processing/LiBa/LiBa_Box2/BMS_CellTemperature/Subsystem5 ==
  byte2 : Inport
  C_LB_BMS_CellTemperature_Timeout : Inport  Port=2
  Bus Creator : BusCreator  Inputs=3
  Constant : Constant  OutDataTypeStr=single
  Constant1 : Constant  Value=0  OutDataTypeStr=single
  Constant2 : Constant  Value=0  OutDataTypeStr=single
  Constant3 : Constant  Value=255  OutDataTypeStr=single
  Constant4 : Constant  Value=0  OutDataTypeStr=single
  Lib_InputProcessing+SafeValueSelector_Data : Library_DataProcessing_v1_1/Lib_InputProcessing+SafeValueSelector_Data  SystemSampleTime=-1  VariantActivationTime=update diagram  Latency=0  AutoFrameSizeCalculation=off
  IP_LB_BMS_ACT_Cel_T_Max_Cel_DataBus : Outport
  wires:
  C_LB_BMS_CellTemperature_Timeout/1 -> Lib_InputProcessing+SafeValueSelector_Data/2
  Bus Creator/1 -> IP_LB_BMS_ACT_Cel_T_Max_Cel_DataBus/1  "IP_LB_BMS_ACT_Cel_T_Max_Cel_DataBus"
  Lib_InputProcessing+SafeValueSelector_Data/1 -> Bus Creator/1
  Constant/1 -> Lib_InputProcessing+SafeValueSelector_Data/3
  Constant4/1 -> Lib_InputProcessing+SafeValueSelector_Data/7, Lib_InputProcessing+SafeValueSelector_Data/8
  Lib_InputProcessing+SafeValueSelector_Data/2 -> Bus Creator/2
  Constant1/1 -> Lib_InputProcessing+SafeValueSelector_Data/4
  byte2/1 -> Lib_InputProcessing+SafeValueSelector_Data/1
  Lib_InputProcessing+SafeValueSelector_Data/3 -> Bus Creator/3
  Constant3/1 -> Lib_InputProcessing+SafeValueSelector_Data/6
  Constant2/1 -> Lib_InputProcessing+SafeValueSelector_Data/5

== system ChiefMaster_TTC580/ChiefMaster/Input Processing/LiBa/LiBa_Box2/BMS_CellTemperature/Subsystem6 ==
  byte3 : Inport
  C_LB_BMS_CellTemperature_Timeout : Inport  Port=2
  Bus Creator : BusCreator  Inputs=3
  Constant : Constant  OutDataTypeStr=single
  Constant1 : Constant  Value=0  OutDataTypeStr=single
  Constant2 : Constant  Value=0  OutDataTypeStr=single
  Constant3 : Constant  Value=255  OutDataTypeStr=single
  Constant4 : Constant  Value=0  OutDataTypeStr=single
  Lib_InputProcessing+SafeValueSelector_Data : Library_DataProcessing_v1_1/Lib_InputProcessing+SafeValueSelector_Data  SystemSampleTime=-1  VariantActivationTime=update diagram  Latency=0  AutoFrameSizeCalculation=off
  IP_LB_BMS_ACT_Cel_V_Max_Cel_DataBus : Outport
  wires:
  Constant2/1 -> Lib_InputProcessing+SafeValueSelector_Data/5
  Constant3/1 -> Lib_InputProcessing+SafeValueSelector_Data/6
  Lib_InputProcessing+SafeValueSelector_Data/3 -> Bus Creator/3
  byte3/1 -> Lib_InputProcessing+SafeValueSelector_Data/1
  Constant1/1 -> Lib_InputProcessing+SafeValueSelector_Data/4
  Lib_InputProcessing+SafeValueSelector_Data/2 -> Bus Creator/2
  Constant4/1 -> Lib_InputProcessing+SafeValueSelector_Data/8, Lib_InputProcessing+SafeValueSelector_Data/7
  Constant/1 -> Lib_InputProcessing+SafeValueSelector_Data/3
  Lib_InputProcessing+SafeValueSelector_Data/1 -> Bus Creator/1
  Bus Creator/1 -> IP_LB_BMS_ACT_Cel_V_Max_Cel_DataBus/1  "IP_LB_BMS_ACT_Cel_T_Max_CMU_DataBus"
  C_LB_BMS_CellTemperature_Timeout/1 -> Lib_InputProcessing+SafeValueSelector_Data/2

== system ChiefMaster_TTC580/ChiefMaster/Input Processing/LiBa/LiBa_Box2/BMS_CellVoltage01/Subsystem ==
  byte0 : Inport
  byte1 : Inport  Port=2
  C_LB_CellVoltage01_Timeout : Inport  Port=3
  Bus Creator : BusCreator  Inputs=3
  Constant : Constant  Value=0.1  OutDataTypeStr=single
  Constant1 : Constant  Value=0  OutDataTypeStr=single
  Constant2 : Constant  Value=0  OutDataTypeStr=single
  Constant3 : Constant  Value=6553.5  OutDataTypeStr=single
  Constant4 : Constant  Value=0  OutDataTypeStr=single
  Lib_2byte_ArthConcat : Library_DataProcessing_v1_1/Lib_2byte_ArthConcat  SystemSampleTime=-1  VariantActivationTime=update diagram  Latency=0  AutoFrameSizeCalculation=off
  Lib_InputProcessing+SafeValueSelector_Data : Library_DataProcessing_v1_1/Lib_InputProcessing+SafeValueSelector_Data  SystemSampleTime=-1  VariantActivationTime=update diagram  Latency=0  AutoFrameSizeCalculation=off
  IP_LB_BMS_ACT_Cel_mV_Min_DataBus : Outport
  wires:
  byte0/1 -> Lib_2byte_ArthConcat/1
  byte1/1 -> Lib_2byte_ArthConcat/2
  Lib_2byte_ArthConcat/1 -> Lib_InputProcessing+SafeValueSelector_Data/1
  C_LB_CellVoltage01_Timeout/1 -> Lib_InputProcessing+SafeValueSelector_Data/2
  Lib_InputProcessing+SafeValueSelector_Data/1 -> Bus Creator/1
  Lib_InputProcessing+SafeValueSelector_Data/2 -> Bus Creator/2
  Lib_InputProcessing+SafeValueSelector_Data/3 -> Bus Creator/3
  Bus Creator/1 -> IP_LB_BMS_ACT_Cel_mV_Min_DataBus/1  "IP_LB_BMS_ACT_Cel_mV_Min_DataBus"
  Constant/1 -> Lib_InputProcessing+SafeValueSelector_Data/3
  Constant1/1 -> Lib_InputProcessing+SafeValueSelector_Data/4
  Constant2/1 -> Lib_InputProcessing+SafeValueSelector_Data/5
  Constant3/1 -> Lib_InputProcessing+SafeValueSelector_Data/6
  Constant4/1 -> Lib_InputProcessing+SafeValueSelector_Data/8, Lib_InputProcessing+SafeValueSelector_Data/7

== system ChiefMaster_TTC580/ChiefMaster/Input Processing/LiBa/LiBa_Box2/BMS_CellVoltage01/Subsystem1 ==
  byte2 : Inport
  byte3 : Inport  Port=2
  C_LB_CellVoltage01_Timeout : Inport  Port=3
  Bus Creator : BusCreator  Inputs=3
  Constant : Constant  Value=0.1  OutDataTypeStr=single
  Constant1 : Constant  Value=0  OutDataTypeStr=single
  Constant2 : Constant  Value=0  OutDataTypeStr=single
  Constant3 : Constant  Value=6553.5  OutDataTypeStr=single
  Constant4 : Constant  Value=0  OutDataTypeStr=single
  Lib_2byte_ArthConcat : Library_DataProcessing_v1_1/Lib_2byte_ArthConcat  SystemSampleTime=-1  VariantActivationTime=update diagram  Latency=0  AutoFrameSizeCalculation=off
  Lib_InputProcessing+SafeValueSelector_Data : Library_DataProcessing_v1_1/Lib_InputProcessing+SafeValueSelector_Data  SystemSampleTime=-1  VariantActivationTime=update diagram  Latency=0  AutoFrameSizeCalculation=off
  IP_LB_BMS_ACT_Cel_mV_AVG_DataBus : Outport
  wires:
  Constant4/1 -> Lib_InputProcessing+SafeValueSelector_Data/8, Lib_InputProcessing+SafeValueSelector_Data/7
  Lib_2byte_ArthConcat/1 -> Lib_InputProcessing+SafeValueSelector_Data/1
  Constant1/1 -> Lib_InputProcessing+SafeValueSelector_Data/4
  Lib_InputProcessing+SafeValueSelector_Data/1 -> Bus Creator/1
  Constant/1 -> Lib_InputProcessing+SafeValueSelector_Data/3
  Lib_InputProcessing+SafeValueSelector_Data/2 -> Bus Creator/2
  Lib_InputProcessing+SafeValueSelector_Data/3 -> Bus Creator/3
  Constant2/1 -> Lib_InputProcessing+SafeValueSelector_Data/5
  Constant3/1 -> Lib_InputProcessing+SafeValueSelector_Data/6
  byte2/1 -> Lib_2byte_ArthConcat/1
  byte3/1 -> Lib_2byte_ArthConcat/2
  C_LB_CellVoltage01_Timeout/1 -> Lib_InputProcessing+SafeValueSelector_Data/2
  Bus Creator/1 -> IP_LB_BMS_ACT_Cel_mV_AVG_DataBus/1  "IP_LB_BMS_ACT_Cel_mV_AVG_DataBus"

== system ChiefMaster_TTC580/ChiefMaster/Input Processing/LiBa/LiBa_Box2/BMS_CellVoltage01/Subsystem2 ==
  byte4 : Inport
  byte5 : Inport  Port=2
  C_LB_CellVoltage01_Timeout : Inport  Port=3
  Bus Creator : BusCreator  Inputs=3
  Constant : Constant  Value=0.1  OutDataTypeStr=single
  Constant1 : Constant  Value=0  OutDataTypeStr=single
  Constant2 : Constant  Value=0  OutDataTypeStr=single
  Constant3 : Constant  Value=6553.5  OutDataTypeStr=single
  Constant4 : Constant  Value=0  OutDataTypeStr=single
  Lib_2byte_ArthConcat : Library_DataProcessing_v1_1/Lib_2byte_ArthConcat  SystemSampleTime=-1  VariantActivationTime=update diagram  Latency=0  AutoFrameSizeCalculation=off
  Lib_InputProcessing+SafeValueSelector_Data : Library_DataProcessing_v1_1/Lib_InputProcessing+SafeValueSelector_Data  SystemSampleTime=-1  VariantActivationTime=update diagram  Latency=0  AutoFrameSizeCalculation=off
  IP_LB_BMS_ACT_Cel_mV_Max_DataBus : Outport
  wires:
  Constant2/1 -> Lib_InputProcessing+SafeValueSelector_Data/5
  Constant3/1 -> Lib_InputProcessing+SafeValueSelector_Data/6
  Lib_InputProcessing+SafeValueSelector_Data/3 -> Bus Creator/3
  Lib_2byte_ArthConcat/1 -> Lib_InputProcessing+SafeValueSelector_Data/1
  Constant1/1 -> Lib_InputProcessing+SafeValueSelector_Data/4
  Lib_InputProcessing+SafeValueSelector_Data/2 -> Bus Creator/2
  Constant4/1 -> Lib_InputProcessing+SafeValueSelector_Data/8, Lib_InputProcessing+SafeValueSelector_Data/7
  Constant/1 -> Lib_InputProcessing+SafeValueSelector_Data/3
  Lib_InputProcessing+SafeValueSelector_Data/1 -> Bus Creator/1
  Bus Creator/1 -> IP_LB_BMS_ACT_Cel_mV_Max_DataBus/1  "IP_LB_BMS_ACT_Cel_mV_Max_DataBus"
  C_LB_CellVoltage01_Timeout/1 -> Lib_InputProcessing+SafeValueSelector_Data/2
  byte4/1 -> Lib_2byte_ArthConcat/1
  byte5/1 -> Lib_2byte_ArthConcat/2

== system ChiefMaster_TTC580/ChiefMaster/Input Processing/LiBa/LiBa_Box2/BMS_CellVoltageNumber/Subsystem ==
  byte0 : Inport
  C_LB_CellVoltage02_Timeout : Inport  Port=2
  Bus Creator : BusCreator  Inputs=3
  Constant : Constant  OutDataTypeStr=single
  Constant1 : Constant  Value=0  OutDataTypeStr=single
  Constant2 : Constant  Value=0  OutDataTypeStr=single
  Constant3 : Constant  Value=255  OutDataTypeStr=single
  Constant4 : Constant  Value=0  OutDataTypeStr=single
  Lib_InputProcessing+SafeValueSelector_Data : Library_DataProcessing_v1_1/Lib_InputProcessing+SafeValueSelector_Data  SystemSampleTime=-1  VariantActivationTime=update diagram  Latency=0  AutoFrameSizeCalculation=off
  IP_LB_BMS_ACT_Cel_V_Min_Cel_DataBus : Outport
  wires:
  Constant4/1 -> Lib_InputProcessing+SafeValueSelector_Data/7, Lib_InputProcessing+SafeValueSelector_Data/8
  Constant3/1 -> Lib_InputProcessing+SafeValueSelector_Data/6
  Constant2/1 -> Lib_InputProcessing+SafeValueSelector_Data/5
  Constant1/1 -> Lib_InputProcessing+SafeValueSelector_Data/4
  Constant/1 -> Lib_InputProcessing+SafeValueSelector_Data/3
  Bus Creator/1 -> IP_LB_BMS_ACT_Cel_V_Min_Cel_DataBus/1  "IP_LB_BMS_ACT_Cel_V_Min_Cel_DataBus"
  Lib_InputProcessing+SafeValueSelector_Data/3 -> Bus Creator/3
  Lib_InputProcessing+SafeValueSelector_Data/2 -> Bus Creator/2
  Lib_InputProcessing+SafeValueSelector_Data/1 -> Bus Creator/1
  C_LB_CellVoltage02_Timeout/1 -> Lib_InputProcessing+SafeValueSelector_Data/2
  byte0/1 -> Lib_InputProcessing+SafeValueSelector_Data/1

== system ChiefMaster_TTC580/ChiefMaster/Input Processing/LiBa/LiBa_Box2/BMS_CellVoltageNumber/Subsystem1 ==
  byte1 : Inport
  C_LB_CellVoltage02_Timeout : Inport  Port=2
  Bus Creator : BusCreator  Inputs=3
  Constant : Constant  OutDataTypeStr=single
  Constant1 : Constant  Value=0  OutDataTypeStr=single
  Constant2 : Constant  Value=0  OutDataTypeStr=single
  Constant3 : Constant  Value=255  OutDataTypeStr=single
  Constant4 : Constant  Value=0  OutDataTypeStr=single
  Lib_InputProcessing+SafeValueSelector_Data : Library_DataProcessing_v1_1/Lib_InputProcessing+SafeValueSelector_Data  SystemSampleTime=-1  VariantActivationTime=update diagram  Latency=0  AutoFrameSizeCalculation=off
  IP_LB_BMS_ACT_Cel_V_Min_CMU_DataBus : Outport
  wires:
  Bus Creator/1 -> IP_LB_BMS_ACT_Cel_V_Min_CMU_DataBus/1  "IP_LB_BMS_ACT_Cel_V_Min_CMU_DataBus"
  C_LB_CellVoltage02_Timeout/1 -> Lib_InputProcessing+SafeValueSelector_Data/2
  Constant3/1 -> Lib_InputProcessing+SafeValueSelector_Data/6
  Constant2/1 -> Lib_InputProcessing+SafeValueSelector_Data/5
  Lib_InputProcessing+SafeValueSelector_Data/3 -> Bus Creator/3
  Lib_InputProcessing+SafeValueSelector_Data/2 -> Bus Creator/2
  Constant/1 -> Lib_InputProcessing+SafeValueSelector_Data/3
  Lib_InputProcessing+SafeValueSelector_Data/1 -> Bus Creator/1
  Constant1/1 -> Lib_InputProcessing+SafeValueSelector_Data/4
  byte1/1 -> Lib_InputProcessing+SafeValueSelector_Data/1
  Constant4/1 -> Lib_InputProcessing+SafeValueSelector_Data/7, Lib_InputProcessing+SafeValueSelector_Data/8

== system ChiefMaster_TTC580/ChiefMaster/Input Processing/LiBa/LiBa_Box2/BMS_CellVoltageNumber/Subsystem2 ==
  byte2 : Inport
  C_LB_CellVoltage02_Timeout : Inport  Port=2
  Bus Creator : BusCreator  Inputs=3
  Constant : Constant  OutDataTypeStr=single
  Constant1 : Constant  Value=0  OutDataTypeStr=single
  Constant2 : Constant  Value=0  OutDataTypeStr=single
  Constant3 : Constant  Value=255  OutDataTypeStr=single
  Constant4 : Constant  Value=0  OutDataTypeStr=single
  Lib_InputProcessing+SafeValueSelector_Data : Library_DataProcessing_v1_1/Lib_InputProcessing+SafeValueSelector_Data  SystemSampleTime=-1  VariantActivationTime=update diagram  Latency=0  AutoFrameSizeCalculation=off
  IP_LB_BMS_ACT_Cel_V_Max_Cel_DataBus : Outport
  wires:
  C_LB_CellVoltage02_Timeout/1 -> Lib_InputProcessing+SafeValueSelector_Data/2
  Bus Creator/1 -> IP_LB_BMS_ACT_Cel_V_Max_Cel_DataBus/1  "IP_LB_BMS_ACT_Cel_V_Max_Cel_DataBus"
  Lib_InputProcessing+SafeValueSelector_Data/1 -> Bus Creator/1
  Constant/1 -> Lib_InputProcessing+SafeValueSelector_Data/3
  Constant4/1 -> Lib_InputProcessing+SafeValueSelector_Data/7, Lib_InputProcessing+SafeValueSelector_Data/8
  Lib_InputProcessing+SafeValueSelector_Data/2 -> Bus Creator/2
  Constant1/1 -> Lib_InputProcessing+SafeValueSelector_Data/4
  byte2/1 -> Lib_InputProcessing+SafeValueSelector_Data/1
  Lib_InputProcessing+SafeValueSelector_Data/3 -> Bus Creator/3
  Constant3/1 -> Lib_InputProcessing+SafeValueSelector_Data/6
  Constant2/1 -> Lib_InputProcessing+SafeValueSelector_Data/5
